simulink model "rtdemoMLEP"  (Simulink 7.7)
settings: Solver=ode4  StartTime=0.0  StopTime=inf  FixedStep=1e-6  RelTol=1e-3
libraries: opal_lib x4, rtlab x2, mlepBlockset x1, simulink x1
Description:
  | Model of a simple control system for use iin training.
settings Model: Creator=Paul Baracos  LastModifiedBy=wbernal  BufferReuse=off
settings DataIOCC: SaveOutput=off  SaveTime=off  SignalLoggingName=sigsOut
settings OptimizationCC: BlockReduction=off  BooleanDataType=off  InlineInvariantSignals=on  OptimizeBlockIOStorage=off  BufferReuse=off  ExpressionFolding=off  LocalBlockOutputs=off  InitFltsAndDblsToZero=on
settings DebuggingCC: SaveWithParameterizedLinksMsg=none  SignalResolutionControl=TryResolveAllWithWarning  SolverPrmCheckMsg=none  MultiTaskDSMMsg=warning  MultiTaskCondExecSysMsg=none  StrictBusMsg=None
settings HardwareCC: TargetUnknown=on
settings RTWCC: IncludeERTFirstTime=on
settings GRTTargetCC: TargetFcnLib=ansi_tfl_tmw.mat

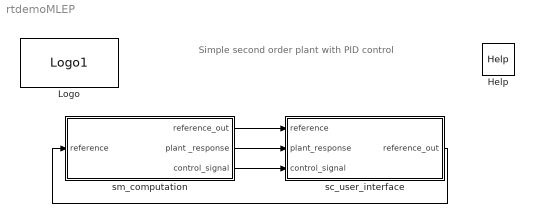
== system rtdemoMLEP ==
  note: Simple second order plant with PID control
  Help : opal_lib/Help  SystemSampleTime=-1  docfile=../help/help.html
  Logo : opal_lib/Logo1  SystemSampleTime=-1
  sc_user_interface : Subsystem
  sm_computation : Subsystem
  wires:
  sc_user_interface/1(reference_out) -> sm_computation/1(reference)
  sm_computation/3(control_signal) -> sc_user_interface/3(control_signal)
  sm_computation/2(plant _response) -> sc_user_interface/2(plant_response)
  sm_computation/1(reference_out) -> sc_user_interface/1(reference)

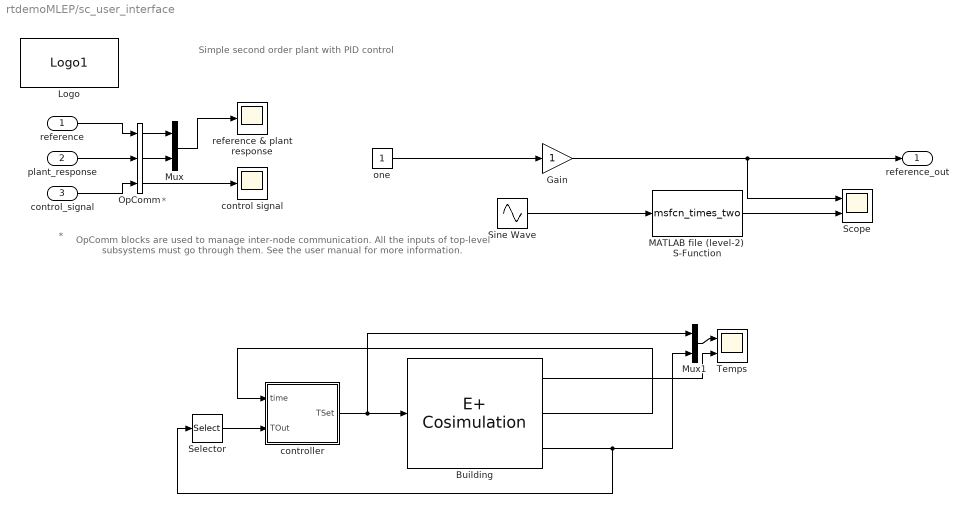
== system rtdemoMLEP/sc_user_interface ==
  note: Simple second order plant with PID control
  note: OpComm blocks are used to manage inter-node communication. All the inputs of top-level
      | subsystems must go through them. See the user manual for more information.
  note: *
  note: *
  reference : Inport
  plant_response : Inport  Port=2
  control_signal : Inport  Port=3
  Building : mlepBlockset/E+ Cosimulation  progname='C:\EnergyPlusV8-0-0-mlep\RunEPlus.bat'  modelfile='SmOffPSZ'  weatherfile='USA_IL_Chicago-OHare.Intl.AP.725300_TMY3'  workdir=''  timeout=60000  port=0  host=''  bcvtbdir='U:\MLE+\mlep_v1.1\MLE+\bcvtb'  deltaT=1e-6  noutputd=2
  Gain : Gain
  Logo : opal_lib/Logo1  SystemSampleTime=-1
  MATLAB file (level-2)  S-Function : M-S-Function  FunctionName=msfcn_times_two
      mask Type: S-function: msfcn_times_two
      mask Description: This is a level-2 MATLAB file S-function which multiply input by two.
      mask Display:
      | plot([0 1 2 3 4 5 6 5 4 3 2 1 0 0],[0 .5 1 1.5 2 2.5 3 3.5 4 4.5 5 5.5 6 0]);
      | disp('2      ');
  Mux : Mux  Inputs=2
  Mux1 : Mux  Inputs=2
  OpComm : rtlab/OpComm  SystemSampleTime=-1  nbport=3  groupe_acq=1  subsys_rate=0  st=0  Synchronization=on  Interpolation=on  Threshold=1.0  Missed_Data=off  Sim_Time=off  Samples=off  dynSigOut=off  from_console=0  warning_done=off  writeOpCommFile=off  Offset=off
  Scope : Scope  NumInputPorts=2
      settings: TickLabels=on  YMin=0.95~-2  YMax=1.05~2
  Selector : Selector  InputPortWidth=2  IndexOptions=Index vector (dialog)  Indices=[1]  OutputSizes=1
  Sine Wave : Sin  SampleTime=0
  Temps : Scope  NumInputPorts=2
      settings: YMin=16~1  YMax=30~1
  control signal : Scope
      settings: YMin=-200  YMax=200  SaveName=controlSignal
  controller : Subsystem
  one : Constant
  reference & plant response : Scope
      settings: Tag=op_tm_save_it  TimeRange=10  YMin=0  YMax=160  SaveName=referenceAndPlant
  reference_out : Outport
  wires:
  Mux/1 -> reference & plant response/1
  reference/1 -> OpComm/1
  control_signal/1 -> OpComm/3
  plant_response/1 -> OpComm/2
  OpComm/1 -> Mux/1
  OpComm/2 -> Mux/2
  OpComm/3 -> control signal/1
  one/1 -> Gain/1
  Sine Wave/1 -> MATLAB file (level-2)  S-Function/1
  MATLAB file (level-2)  S-Function/1 -> Scope/2
  Gain/1 -> reference_out/1, Scope/1
  controller/1(TSet) -> Mux1/1, Building/1
  Building/2 -> controller/1(time)
  Building/3 -> Mux1/2, Selector/1
  Mux1/1 -> Temps/1
  Selector/1 -> controller/2(TOut)
  Building/1 -> Temps/2

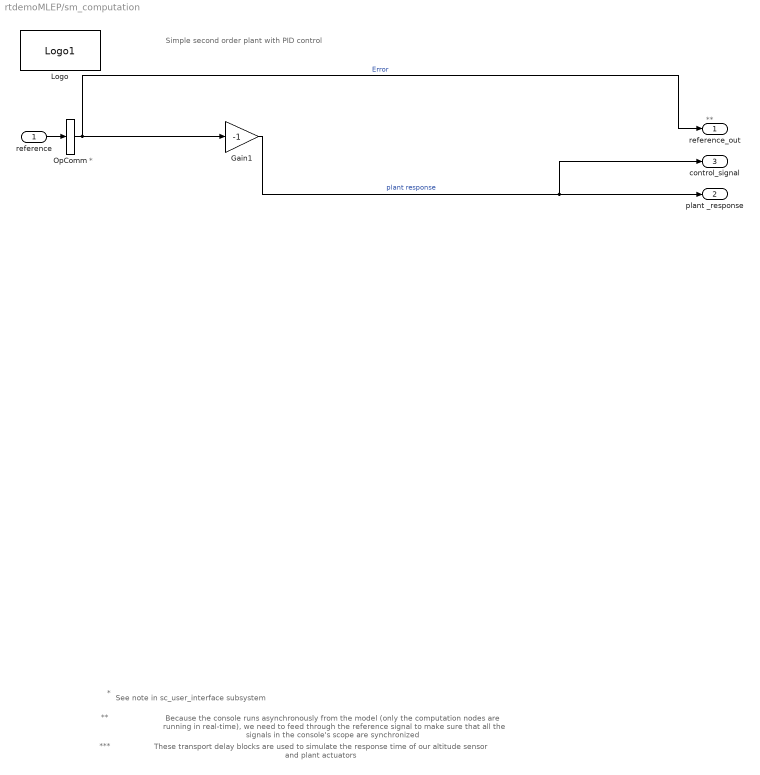
== system rtdemoMLEP/sm_computation ==
  note: Simple second order plant with PID control
  note: Because the console runs asynchronously from the model (only the computation nodes are running in real-time), we
      | need to feed through the reference signal to make sure that all the signals in the console's scope are synchronized
  note: **
  note: **
  note: *
  note: See note in sc_user_interface subsystem
  note: *
  note: These transport delay blocks are used to simulate the response time of our altitude sensor and plant actuators
  note: ***
  reference : Inport
  Gain1 : Gain  Gain=-1  SaturateOnIntegerOverflow=on  OutDataTypeStr=Inherit: Same as input  ParamDataTypeStr=Inherit: Same as input
  Logo : opal_lib/Logo1  SystemSampleTime=-1
  OpComm : rtlab/OpComm  SystemSampleTime=-1  nbport=1  groupe_acq=1  subsys_rate=0  st=0  Synchronization=on  Interpolation=on  Threshold=1.0  Missed_Data=off  Sim_Time=off  Samples=off  dynSigOut=off  from_console=1  warning_done=off  writeOpCommFile=off  Offset=off
  reference_out : Outport
  plant _response : Outport  Port=2
  control_signal : Outport  Port=3
  wires:
  reference/1 -> OpComm/1
  OpComm/1 -> reference_out/1, Gain1/1  "Error"
  Gain1/1 -> plant _response/1, control_signal/1  "plant response"

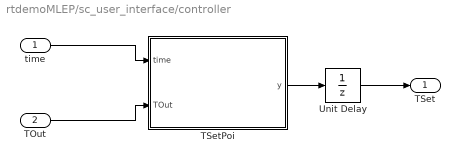
== system rtdemoMLEP/sc_user_interface/controller ==
  time : Inport
  TOut : Inport  Port=2
  TSetPoi : Subsystem
  Unit Delay : UnitDelay  X0=[20, 25]  SampleTime=-1
  TSet : Outport
  wires:
  time/1 -> TSetPoi/1(time)
  TOut/1 -> TSetPoi/2(TOut)
  Unit Delay/1 -> TSet/1
  TSetPoi/1(y) -> Unit Delay/1

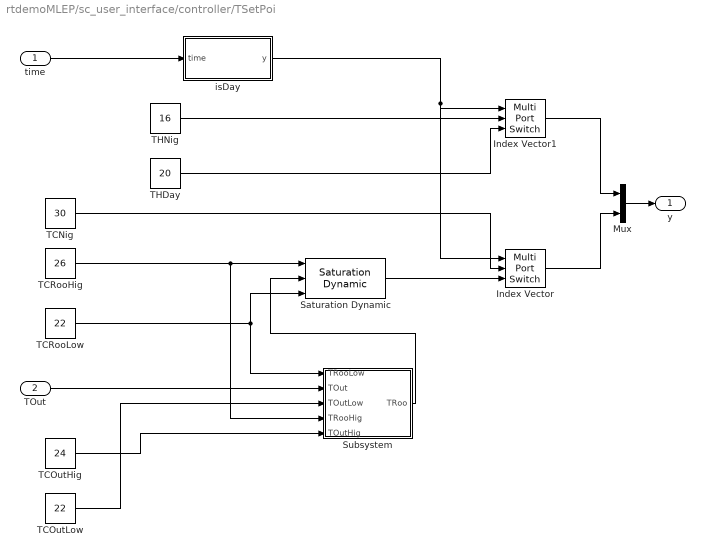
== system rtdemoMLEP/sc_user_interface/controller/TSetPoi ==
  time : Inport
  TOut : Inport  Port=2
  Index Vector : MultiPortSwitch  DataPortOrder=Zero-based contiguous  Inputs=2  zeroidx=on
  Index Vector1 : MultiPortSwitch  DataPortOrder=Zero-based contiguous  Inputs=2  zeroidx=on
  Mux : Mux  Inputs=2
  Saturation Dynamic : simulink/Discontinuities/Saturation Dynamic  SystemSampleTime=-1  OutMin=[]  OutMax=[]  OutDataTypeStr=Inherit: Same as second input  OutDataType=sfix(16)  OutScaling=2^-10  DoSatur=off
  Subsystem : Subsystem
  TCNig : Constant  Value=30
  TCOutHig : Constant  Value=24
  TCOutLow : Constant  Value=22
  TCRooHig : Constant  Value=26
  TCRooLow : Constant  Value=22
  THDay : Constant  Value=20
  THNig : Constant  Value=16
  isDay : Subsystem
  y : Outport
  wires:
  TOut/1 -> Subsystem/2(TOut)
  TCOutLow/1 -> Subsystem/3(TOutLow)
  TCOutHig/1 -> Subsystem/5(TOutHig)
  TCRooHig/1 -> Saturation Dynamic/1, Subsystem/4(TRooHig)
  TCRooLow/1 -> Saturation Dynamic/3, Subsystem/1(TRooLow)
  time/1 -> isDay/1(time)
  isDay/1(y) -> Index Vector/1, Index Vector1/1
  TCNig/1 -> Index Vector/2
  Subsystem/1(TRoo) -> Saturation Dynamic/2
  Saturation Dynamic/1 -> Index Vector/3
  THNig/1 -> Index Vector1/2
  THDay/1 -> Index Vector1/3
  Index Vector1/1 -> Mux/1
  Index Vector/1 -> Mux/2
  Mux/1 -> y/1

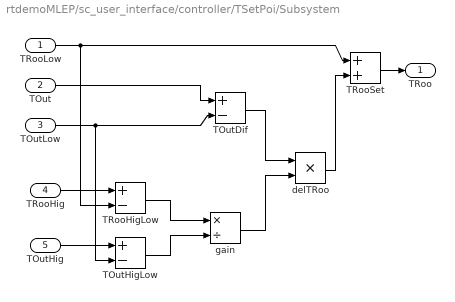
== system rtdemoMLEP/sc_user_interface/controller/TSetPoi/Subsystem ==
  TRooLow : Inport
  TOut : Inport  Port=2
  TOutLow : Inport  Port=3
  TRooHig : Inport  Port=4
  TOutHig : Inport  Port=5
  TOutDif : Sum  Inputs=+-
  TOutHigLow : Sum  Inputs=+-
  TRooHigLow : Sum  Inputs=+-
  TRooSet : Sum
  delTRoo : Product  RndMeth=Zero
  gain : Product  Inputs=*/
  TRoo : Outport
  wires:
  TRooHigLow/1 -> gain/1
  TOutHigLow/1 -> gain/2
  TOutDif/1 -> delTRoo/1
  gain/1 -> delTRoo/2
  delTRoo/1 -> TRooSet/2
  TRooLow/1 -> TRooSet/1, TRooHigLow/2
  TOutLow/1 -> TOutDif/2, TOutHigLow/2
  TRooHig/1 -> TRooHigLow/1
  TOutHig/1 -> TOutHigLow/1
  TRooSet/1 -> TRoo/1
  TOut/1 -> TOutDif/1

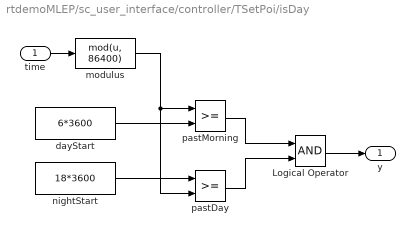
== system rtdemoMLEP/sc_user_interface/controller/TSetPoi/isDay ==
  time : Inport
  Logical Operator : Logic  AllPortsSameDT=off  OutDataTypeStr=boolean
  dayStart : Constant  Value=6*3600
  modulus : MATLABFcn  MATLABFcn=mod(u, 86400)
  nightStart : Constant  Value=18*3600
  pastDay : RelationalOperator  OutDataTypeStr=boolean
  pastMorning : RelationalOperator  OutDataTypeStr=boolean
  y : Outport
  wires:
  time/1 -> modulus/1
  modulus/1 -> pastMorning/1, pastDay/2
  dayStart/1 -> pastMorning/2
  nightStart/1 -> pastDay/1
  pastMorning/1 -> Logical Operator/1
  pastDay/1 -> Logical Operator/2
  Logical Operator/1 -> y/1
